simulink model "Propulsion_simulation"  (R2014b)
settings: Solver=VariableStepAuto  StartTime=0.0  StopTime=100  RelTol=1e-3
values from neighbouring files (symbols this model uses):
  gamma = 1.4    [propulsion_sim1.m]
  P0 = 4000    [propulsion_sim1.m]
  R = 287    [propulsion_sim1.m]
  T0 = 300    [propulsion_sim1.m]
libraries: simulink x1
settings Model: Creator=vvlakshm  LastModifiedBy=shubhamsonawani
settings DataIOCC: LimitDataPoints=off  SaveFormat=Dataset
settings OptimizationCC: UseDivisionForNetSlopeComputation=off  SimCompilerOptimization=off
settings DebuggingCC: SolverPrmCheckMsg=none  FrameProcessingCompatibilityMsg=error
settings HardwareCC: ProdBitPerPointer=64  ProdLargestAtomicFloat=Float  ProdIntDivRoundTo=Zero  ProdEndianess=LittleEndian  ProdWordSize=64  ProdHWDeviceType=Intel->x86-64 (Windows64)
settings ModelReferenceCC: PropagateSignalLabelsOutOfModel=on
settings RTWCC: RTWCompilerOptimization=off
settings ConfigComp: CovMetricSettings=dw  CovHtmlReporting=on  CovSaveCumulativeToWorkspaceVar=on  CovSaveSingleToWorkspaceVar=on  CovExternalEMLEnable=off

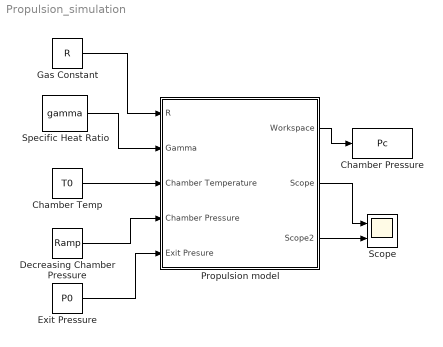
== system Propulsion_simulation ==
  "Chamber Pressure " : ToWorkspace  VariableName=Pc  SaveFormat=Timeseries  SampleTime=-1
  "Chamber Temp " : Constant  Value=T0
  Decreasing Chamber Pressure : simulink/Sources/Ramp  slope=-4635662.65  start=0  X0=9653000
  Exit Pressure : Constant  Value=P0
  Gas Constant : Constant  Value=R
  Propulsion model : Subsystem
  Scope : Scope  NumInputPorts=2
      settings: YMin=29.2042~-5  YMax=750.412~5
  Specific Heat Ratio : Constant  Value=gamma
  wires:
  Specific Heat Ratio/1 -> Propulsion model/2(Gamma)
  Gas Constant/1 -> Propulsion model/1(R)
  Exit Pressure/1 -> Propulsion model/5(Exit Presure)
  "Chamber Temp "/1 -> Propulsion model/3(Chamber Temperature)
  Decreasing Chamber Pressure/1 -> Propulsion model/4(Chamber Pressure)
  Propulsion model/1(Workspace) -> "Chamber Pressure "/1
  Propulsion model/2(Scope) -> Scope/1
  Propulsion model/3(Scope2) -> Scope/2

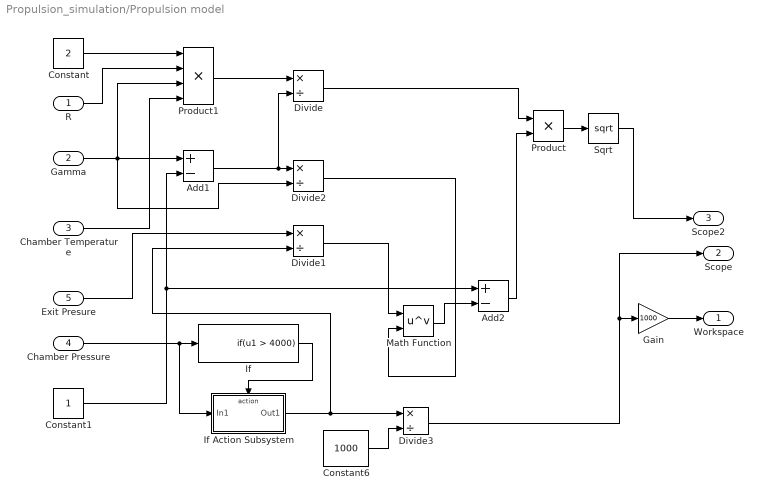
== system Propulsion_simulation/Propulsion model ==
  R : Inport
  Gamma : Inport  Port=2
  Chamber Temperature : Inport  Port=3
  Chamber Pressure : Inport  Port=4
  Exit Presure : Inport  Port=5
  Add1 : Sum  Inputs=+-
  Add2 : Sum  Inputs=+-
  Constant : Constant  Value=2
  Constant1 : Constant
  Constant6 : Constant  Value=1000
  Divide{,1..3} (4 alike) : Product  Inputs=*/
  Gain : Gain  Gain=1000
  If : If  IfExpression=u1 > 4000  ShowElse=off
  If Action Subsystem : Subsystem  TreatAsAtomicUnit=on
  Math Function : Math  Operator=pow  OutputSignalType=real  SaturateOnIntegerOverflow=on
  Product : Product
  Product1 : Product  Inputs=4
  Sqrt : Sqrt  SaturateOnIntegerOverflow=on
  Workspace : Outport
  Scope : Outport  Port=2
  Scope2 : Outport  Port=3
  wires:
  Product1/1 -> Divide/1
  Add1/1 -> Divide2/1, Divide/2
  Divide/1 -> Product/1
  Divide1/1 -> Math Function/1
  Divide2/1 -> Math Function/2
  Product/1 -> Sqrt/1
  Math Function/1 -> Add2/2
  Add2/1 -> Product/2
  If/1 -> If Action Subsystem/Action
  If Action Subsystem/1(Out1) -> Divide1/2, Divide3/1
  Sqrt/1 -> Scope2/1
  Constant6/1 -> Divide3/2
  Divide3/1 -> Scope/1, Gain/1
  Gain/1 -> Workspace/1
  Constant/1 -> Product1/1
  R/1 -> Product1/2
  Gamma/1 -> Divide2/2, Product1/3, Add1/1
  Chamber Temperature/1 -> Product1/4
  Constant1/1 -> Add1/2, Add2/1
  Exit Presure/1 -> Divide1/1
  Chamber Pressure/1 -> If/1, If Action Subsystem/1(In1)

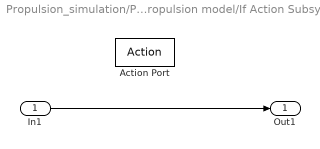
== system Propulsion_simulation/Propulsion model/If Action Subsystem ==
  In1 : Inport
  Action Port : ActionPort  ActionType=then
  Out1 : Outport
  wires:
  In1/1 -> Out1/1
